simulink model "Reshape_ColumnVector"  (R2017b)
settings: Solver=FixedStepAuto  StartTime=0.0  StopTime=10.0  FixedStep=0.1  RelTol=1e-3  EnableMultiTasking=on
model workspace (MAT data in the model file):
  A = reshape([0.616044676147 0.473288848903 0.351659507063 0.830828627896 0.585264091153 0.549723608291 0.91719366383 0.28583901882 0.757200229111 0.753729094278 0.380445846975 0.567821640725 0.0758542895631 0.0539501186666 0.530797553009 0.779167230102 0.934010684229 0.129906208474 0.568823660872 0.469390641058 0.0119020695012 0.337122644399 0.162182308193 0.794284540684 0.311215042045 0.528533135506 0.1656487295 0.601981941402 0.26297128454 0.654079098477 0.68921450314 0.748151592824 0.450541598502 0.0838213779969 0.228976968717 0.913337361502 0.152378018969 0.82581697749 0.53834243526 0.996134716627 0.0781755287532 0.442678269775 0.106652770181 0.961898080855 0.00463422413407 0.774910464712 0.817303220653 0.868694705364], [2 3 4 2])
settings Model: Creator=ktrinh  LastModifiedBy=hbourbou
settings OptimizationCC: LifeSpan=inf
settings DebuggingCC: SFUnexpectedBacktrackingDiag=warning  SFNoUnconditionalDefaultTransitionDiag=warning  SFExecutionAtInitializationDiag=none
settings HardwareCC: ProdBitPerSizeT=32  ProdBitPerPtrDiffT=32  ProdWordSize=32  ProdHWDeviceType=Specified
settings CodeAppCC: StateflowObjectComments=on
settings GRTTargetCC: TargetLangStandard=C89/C90 (ANSI)  GeneratePreprocessorConditionals=Disable all
settings ConfigComp: CovMetricSettings=dw  CovHtmlReporting=on  CovSaveCumulativeToWorkspaceVar=on  CovSaveSingleToWorkspaceVar=on  CovExternalEMLEnable=off

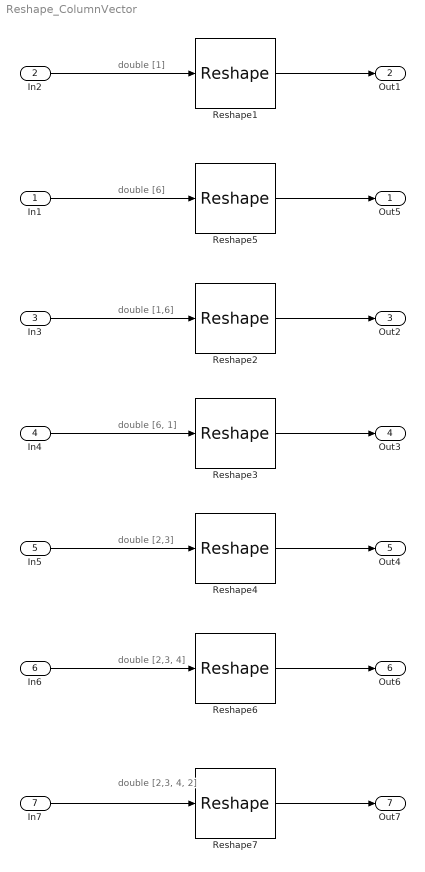
== system Reshape_ColumnVector ==
  note: double [6]
  note: double [1]
  note: double [1,6]
  note: double [6, 1]
  note: double [2,3]
  note: double [2,3, 4]
  note: double [2,3, 4, 2]
  In1 : Inport  PortDimensions=[6]
  In2 : Inport  Port=2
  In3 : Inport  Port=3  PortDimensions=[1,6]
  In4 : Inport  Port=4  PortDimensions=[6 1]
  In5 : Inport  Port=5  PortDimensions=[2 3]
  In6 : Inport  Port=6  PortDimensions=[2 3 4]
  In7 : Inport  Port=7  PortDimensions=[2 3 4 2]
  Reshape{1..7} (7 alike) : Reshape  OutputDimensionality=Column vector (2-D)
  Out5 : Outport
  Out1 : Outport  Port=2
  Out2 : Outport  Port=3
  Out3 : Outport  Port=4
  Out4 : Outport  Port=5
  Out6 : Outport  Port=6
  Out7 : Outport  Port=7
  wires:
  In1/1 -> Reshape5/1
  Reshape5/1 -> Out5/1
  In2/1 -> Reshape1/1
  Reshape1/1 -> Out1/1
  In3/1 -> Reshape2/1
  Reshape2/1 -> Out2/1
  In4/1 -> Reshape3/1
  Reshape3/1 -> Out3/1
  In5/1 -> Reshape4/1
  Reshape4/1 -> Out4/1
  In6/1 -> Reshape6/1
  Reshape6/1 -> Out6/1
  In7/1 -> Reshape7/1
  Reshape7/1 -> Out7/1
